simulink model "newBLDCmodel_r2018a"  (R2018a)
settings: Solver=VariableStepAuto  StartTime=0.0  StopTime=10  MaxStep=.001  RelTol=1e-3
libraries: simulink x1
settings Model: Creator=tdarrah  LastModifiedBy=tdarrah
settings SolverCC: InitialStep=.001  ShapePreserveControl=EnableAll
settings CodeAppCC: StateflowObjectComments=on

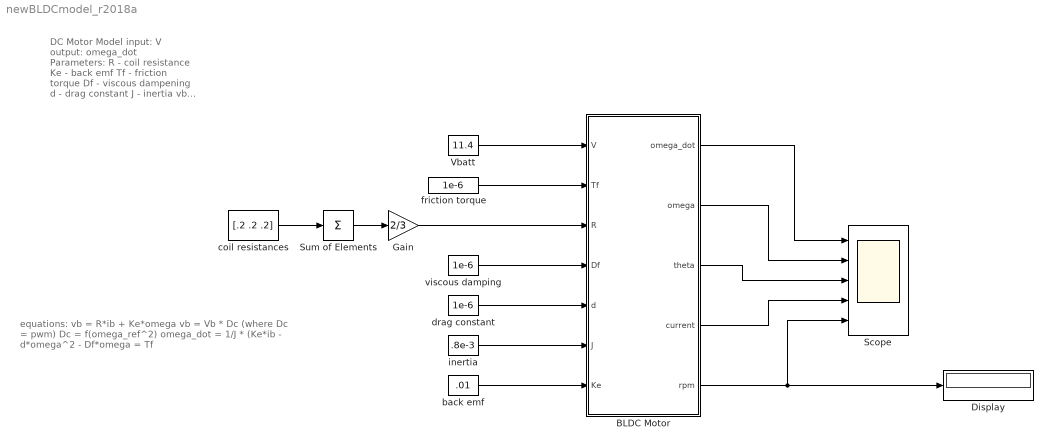
== system newBLDCmodel_r2018a ==
  note: equations:
      |
      | vb = R*ib + Ke*omega
      | vb = Vb * Dc  (where Dc = pwm)
      | Dc = f(omega_ref^2)
      |
      | omega_dot = 1/J * (Ke*ib - d*omega^2 - Df*omega = Tf
  note: DC Motor Model
      |
      | input:
      | V
      |
      | output:
      | omega_dot
      |
      | Parameters:
      | R   - coil resistance
      | Ke - back emf
      | Tf  - friction torque
      | Df  - viscous dampening
      | d   - drag constant
      | J   - inertia
      | vb - average battery voltage
      | ib  - average battery current
  BLDC Motor : Subsystem
  Display : Display
  Gain : Gain  Gain=2/3
  Scope : Scope  NumInputPorts=5
  Sum of Elements : Sum  Inputs=+
  Vbatt : Constant  Value=11.4
  back emf : Constant  Value=.01
  coil resistances : Constant  Value=[.2 .2 .2]
  drag constant : Constant  Value=1e-6
  friction torque : Constant  Value=1e-6
  inertia : Constant  Value=.8e-3
  viscous damping : Constant  Value=1e-6
  wires:
  BLDC Motor/2(omega) -> Scope/2
  BLDC Motor/3(theta) -> Scope/3
  BLDC Motor/5(rpm) -> Scope/5, Display/1
  BLDC Motor/4(current) -> Scope/4
  BLDC Motor/1(omega_dot) -> Scope/1
  Sum of Elements/1 -> Gain/1
  coil resistances/1 -> Sum of Elements/1
  Gain/1 -> BLDC Motor/3(R)
  Vbatt/1 -> BLDC Motor/1(V)
  friction torque/1 -> BLDC Motor/2(Tf)
  back emf/1 -> BLDC Motor/7(Ke)
  viscous damping/1 -> BLDC Motor/4(Df)
  drag constant/1 -> BLDC Motor/5(d)
  inertia/1 -> BLDC Motor/6(J)

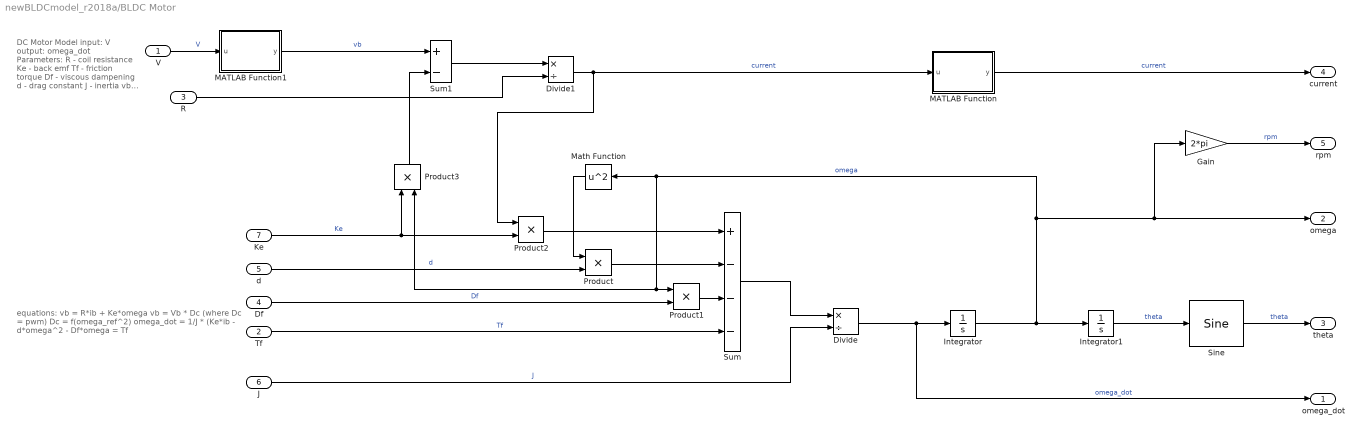
== system newBLDCmodel_r2018a/BLDC Motor ==
  note: DC Motor Model
      |
      | input:
      | V
      |
      | output:
      | omega_dot
      |
      | Parameters:
      | R   - coil resistance
      | Ke - back emf
      | Tf  - friction torque
      | Df  - viscous dampening
      | d   - drag constant
      | J   - inertia
      |
      |
      | vb - average battery voltage
      | ib  - average battery current
  note: equations:
      |
      | vb = R*ib + Ke*omega
      | vb = Vb * Dc  (where Dc = pwm)
      | Dc = f(omega_ref^2)
      |
      | omega_dot = 1/J * (Ke*ib - d*omega^2 - Df*omega = Tf
  V : Inport
  Tf : Inport  Port=2
  R : Inport  Port=3
  Df : Inport  Port=4
  d : Inport  Port=5
  J : Inport  Port=6
  Ke : Inport  Port=7
  Divide : Product  Inputs=*/
  Divide1 : Product  Inputs=*/
  Gain : Gain  Gain=2*pi
  Integrator : Integrator
  Integrator1 : Integrator
  MATLAB Function : MATLAB Function  TreatAsAtomicUnit=on
  MATLAB Function1 : MATLAB Function  TreatAsAtomicUnit=on
  Math Function : Math  Operator=square  SaturateOnIntegerOverflow=on
  Product{,1..3} (4 alike) : Product
  Sine : simulink/Lookup Tables/Sine  Formula=sin(2*pi*u)  NumDataPoints=180  OutputWordLength=16  InternalRulePriority=Speed
      settings: SourceProductName=Simulink
  Sum : Sum  Inputs=+---
  Sum1 : Sum  Inputs=+-
  omega_dot : Outport
  omega : Outport  Port=2
  theta : Outport  Port=3
  current : Outport  Port=4
  rpm : Outport  Port=5
  wires:
  Divide/1 -> omega_dot/1, Integrator/1  "omega_dot"
  Integrator/1 -> Gain/1, omega/1, Math Function/1, Product3/2, Product1/1, Integrator1/1  "omega"
  Integrator1/1 -> Sine/1  "theta"
  Gain/1 -> rpm/1  "rpm"
  Sum/1 -> Divide/1
  J/1 -> Divide/2  "J"
  d/1 -> Product/2  "d"
  Product/1 -> Sum/2
  Math Function/1 -> Product/1
  Product1/1 -> Sum/3
  Df/1 -> Product1/2  "Df"
  Tf/1 -> Sum/4  "Tf"
  Ke/1 -> Product3/1, Product2/2  "Ke"
  Product2/1 -> Sum/1
  Divide1/1 -> Product2/1, MATLAB Function/1(u)  "current"
  V/1 -> MATLAB Function1/1(u)  "V"
  Product3/1 -> Sum1/2
  MATLAB Function/1(y) -> current/1  "current"
  MATLAB Function1/1(y) -> Sum1/1  "vb"
  Sum1/1 -> Divide1/1
  R/1 -> Divide1/2
  Sine/1 -> theta/1  "theta"

== matlab function newBLDCmodel_r2018a/BLDC Motor/MATLAB Function1 ==
  data: u input; y output
function y = Dc(u)

y = 1*u;

== matlab function newBLDCmodel_r2018a/BLDC Motor/MATLAB Function ==
  data: u input; y output
function y = Dc(u)

y = 1*u;
